simulink model "visual_line_follower_sac_lyapunov_prevlat_20260707_113326"  (R2026a)
settings: Solver=FixedStepDiscrete  StopTime=50  FixedStep=MJ_StepTime  EnableMultiTasking=on
InitFcn:
  | run(fullfile(fileparts(get_param(bdroot,"FileName")),"runtime","configure_turtlebot3_visual_line_follower_paths.m"));
model workspace (MAT data in the model file):
  BaseLinearSpeed = 20
  BaseSpeedScale = 0.03
  Kd_Line = 0.35
  Ki_Line = 0
  Kp_Line = 5
  LocalPath_CurvatureGain = 0.04
  LocalPath_HeadingGain = 0.35
  LocalPath_LateralGain = 0.6
  LocalPath_LookaheadDistance = 0.72
  LocalPath_NumPoints = 30
  LocalPath_ROIFraction = 0.1
  MJ_StepTime = 0.002
  MJ_TargetLateralPosition = 0
  MaxAngularSpeed = 1.5
  MaxWheelSpeed = 25
  N_Line = 20
  OriginBot_ErrorScale = 500
  OriginBot_MaxSaturation = 0.3
  OriginBot_MinBrightness = 70
  OriginBot_MinPixels = 30
  OriginBot_ROIHeight = 45
  OriginBot_ROIStartFraction = 0.72
  SAC_Beta = 3
  SAC_Done_Steps = 100
  SAC_Eps = 0.01
  SAC_K_inv = 0.4
  SAC_Lambda = 0.5
  SAC_MaxDeltaOmega = 1
  SAC_P_Lost = 1
  SAC_Q = 1
  SAC_Q_e = 1
  SAC_Q_h = 1
  SAC_Q_l = 1
  SAC_R = 0.1
  SteeringSign = 1
  TB3_WheelRadius = 0.033
  TB3_WheelSeparation = 0.288
  Ts_Control = 0.05
  Ts_Stop = 10
  Ts_Vision = 0.05
  TurtleBot3MuJoCoMap = "training"
  TurtleBot3MuJoCoScene = ""
undefined symbols (not defined in the file): originbot_line_follower_debug_frame, originbot_local_path_generator
libraries: mjLib x1, slpidlib x1, simulink x1, rllib x1
settings Model: ExtModeTrigDuration=10000  Creator=HP  LastModifiedBy=HP
settings SolverCC: PositivePriorityOrder=on
settings ConfigComp: CovMetricSettings=dswe

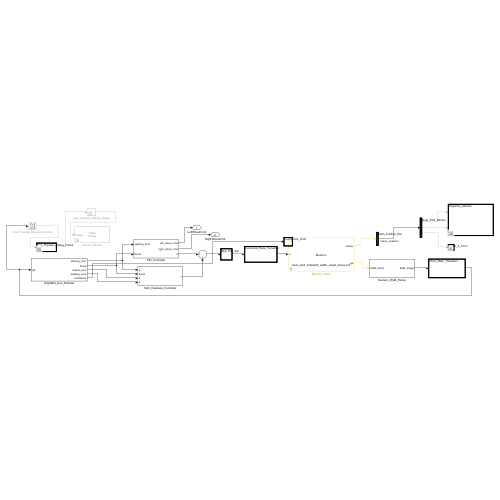
[thumbnail: Simulink's stored preview of the top-level diagram]
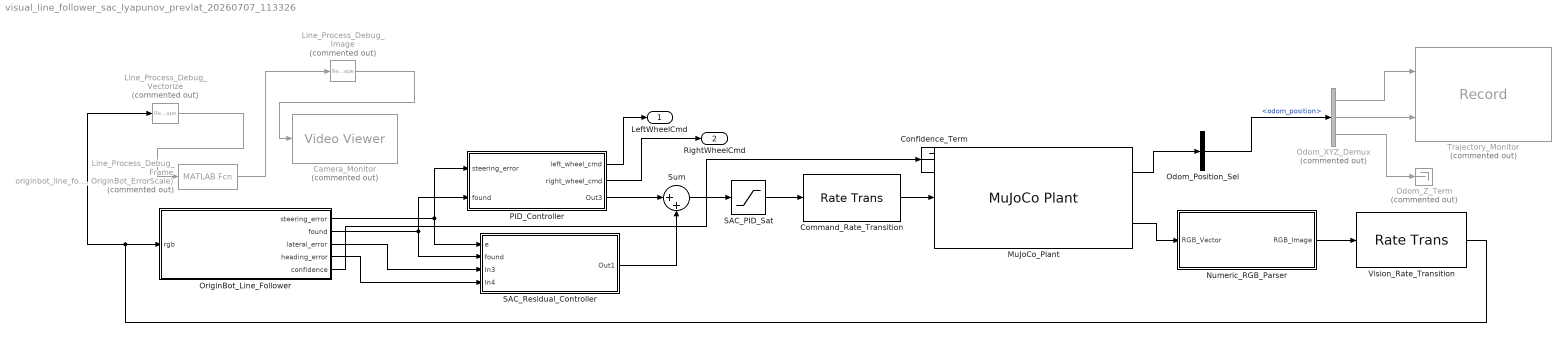
== system visual_line_follower_sac_lyapunov_prevlat_20260707_113326 ==
  Camera_Monitor : VideoViewer  Commented=on  FigPos=[498 692 990 438]
  Command_Rate_Transition : RateTransition  OutPortSampleTime=MJ_StepTime
  Confidence_Term : Terminator
  Line_Process_Debug_Frame : MATLABFcn  Commented=on  MATLABFcn=originbot_line_follower_debug_frame(u, LocalPath_ROIFraction, LocalPath_NumPoints, OriginBot_MinBrightness, OriginBot_MaxSaturation, OriginBot_MinPixels, OriginBot_ErrorScale)
  Line_Process_Debug_Image : Reshape  Commented=on  OutputDimensionality=Customize  OutputDimensions=[480,640,3]
  Line_Process_Debug_Vectorize : Reshape  Commented=on  OutputDimensionality=Column vector (2-D)
  MuJoCo_Plant : mjLib/MuJoCo Plant  controlBus=[]  sensorBus=mj_bus_sensor_7979902499018342666  controlLength=[]  sensorLength=[]  rgbLength=[]  depthLength=[]  sampleTime=0.002  xmlFileRel=D:\final_project\Sheffield\for_getting_started\src\simple_camera_pid\matlab\..\..\..\model\mujoco\turtlebot3\training_oval_track_turtlebot3_waffle_visual_scene.xml  xmlFile=D:\final_project\Sheffield\for_getting_started\src\simple_camera_pid\matlab\..\..\..\model\mujoco\turtlebot3\track_hard_turtlebot3_waffle_visual_scene.xml  renderingType=None  vsync=on  visualFPS=60  zoomLevel=1  znear=0.062275  zfar=311.3772  cameraSampleTime=Ts_Vision  rgbOutOption=on  depthOutOption=off  controlInterfaceType=Vector
      settings: SourceProductName=MuJoCo Simulator
  Numeric_RGB_Parser : Subsystem
  Odom_Position_Sel : BusSelector  OutputSignals=odom_position
  Odom_XYZ_Demux : Demux  Commented=on  Outputs=3
  Odom_Z_Term : Terminator  Commented=on
  OriginBot_Line_Follower : Subsystem
  PID_Controller : Subsystem
  SAC_PID_Sat : Saturate  UpperLimit=[MaxWheelSpeed; MaxWheelSpeed]  LowerLimit=-[MaxWheelSpeed; MaxWheelSpeed]
  SAC_Residual_Controller : Subsystem
  Sum : Sum  Inputs=|++
  Trajectory_Monitor : Record  Commented=on  NumPorts=2.0  FileSettingsInternal="{\"entries\":[{\"content\":{\"excelSettings\":{\"content\":{},\"type\":\"Streamout.ExcelSettings\"},\"parquetSettings\":{\"content\":{},\"type\":\"Streamout.ParquetSettings\"}},\"type\":\"Streamout.FileSettingStorage\",\"uuid\":\"\"}],\"packageUris\":[\"http:\\/\\/schema.mathworks.com\\/mf0\\/streamout_blocks\\/R2020a\"],\"version\":\"1.0\"}"  FrameSettings=[0, 0]  Layout=[1 1]  SignalsInternal="{\"entries\":[{\"content\":{\"signals\":[{\"content\":{\"blockPath\":[],\"dimensions\":[1,1],\"domain\":\"\",\"lineColor\":\"#a2142f\",\"plots\":[ 1 ],\"port\":1,\"signalID\":1,\"signalName\":\"Odom_XYZ_Demux:1\"},\"type\":\"RecordBlkView.Signal\",\"uuid\":\"\"},{\"content\":{\"blockPath\":[],\"dimensions\":[1,1],\"domain\":\"\",\"lineColor\":\"#139fff\",\"plots\":[ 1 ],\"port\":2,\"signalID\":2,\"signalName\":\"Odom_XYZ_Demux:2\"},\"type\":\"RecordBlkView.Signal\",\"uuid\":\"\"}]},\"type\":\"RecordBlkView.InputSignals\",\"uuid\":\"\"}],\"packageUris\":[\"http:\\/\\/schema.mathworks.com\\/mf0\\/streamout_blocks\\/R2020a\"],\"version\":\"1.0\"}"  VisualizationBindings="{\"xyplotplugin\":{\"info\":[{\"series\":[{\"bindingParametersList\":[{\"parameter\":\"X-Axis\",\"signalID\":1,\"signalName\":\"Odom_XYZ_Demux:1\"},{\"parameter\":\"Y-Axis\",\"signalID\":2,\"signalName\":\"Odom_XYZ_Demux:2\"}],\"seriesID\":0}],\"subplotID\":1}]}}"  CompatibilityTag=XY  st=-1
  Vision_Rate_Transition : RateTransition  OutPortSampleTime=Ts_Vision
  LeftWheelCmd : Outport
  RightWheelCmd : Outport  Port=2
  wires:
  Line_Process_Debug_Frame/1 -> Line_Process_Debug_Image/1
  Vision_Rate_Transition/1 -> OriginBot_Line_Follower/1(rgb), Line_Process_Debug_Vectorize/1
  PID_Controller/1(left_wheel_cmd) -> LeftWheelCmd/1
  Line_Process_Debug_Vectorize/1 -> Line_Process_Debug_Frame/1
  MuJoCo_Plant/2 -> Numeric_RGB_Parser/1(RGB_Vector)
  OriginBot_Line_Follower/2(found) -> PID_Controller/2(found), SAC_Residual_Controller/2(found)
  OriginBot_Line_Follower/1(steering_error) -> PID_Controller/1(steering_error), SAC_Residual_Controller/1(e)
  Command_Rate_Transition/1 -> MuJoCo_Plant/1
  PID_Controller/2(right_wheel_cmd) -> RightWheelCmd/1
  Line_Process_Debug_Image/1 -> Camera_Monitor/1
  Numeric_RGB_Parser/1(RGB_Image) -> Vision_Rate_Transition/1
  OriginBot_Line_Follower/3(lateral_error) -> SAC_Residual_Controller/3(In3)
  OriginBot_Line_Follower/4(heading_error) -> SAC_Residual_Controller/4(In4)
  PID_Controller/3(Out3) -> Sum/1
  SAC_Residual_Controller/1(Out1) -> Sum/2
  Sum/1 -> SAC_PID_Sat/1
  SAC_PID_Sat/1 -> Command_Rate_Transition/1
  MuJoCo_Plant/1 -> Odom_Position_Sel/1
  Odom_Position_Sel/1 -> Odom_XYZ_Demux/1  "<odom_position>"
  Odom_XYZ_Demux/1 -> Trajectory_Monitor/1
  Odom_XYZ_Demux/2 -> Trajectory_Monitor/2
  Odom_XYZ_Demux/3 -> Odom_Z_Term/1
  OriginBot_Line_Follower/5(confidence) -> Confidence_Term/1

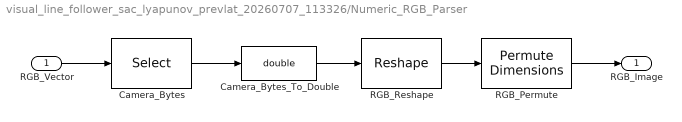
== system visual_line_follower_sac_lyapunov_prevlat_20260707_113326/Numeric_RGB_Parser ==
  RGB_Vector : Inport
  Camera_Bytes : Selector  InputPortWidth=921601  IndexOptions=Index vector (dialog)  Indices=1:921600  OutputSizes=1
  Camera_Bytes_To_Double : DataTypeConversion  OutDataTypeStr=double
  RGB_Permute : PermuteDimensions  Order=[3 2 1]
  RGB_Reshape : Reshape  OutputDimensionality=Customize  OutputDimensions=[3,640,480]
  RGB_Image : Outport
  wires:
  Camera_Bytes_To_Double/1 -> RGB_Reshape/1
  RGB_Permute/1 -> RGB_Image/1
  RGB_Reshape/1 -> RGB_Permute/1
  Camera_Bytes/1 -> Camera_Bytes_To_Double/1
  RGB_Vector/1 -> Camera_Bytes/1

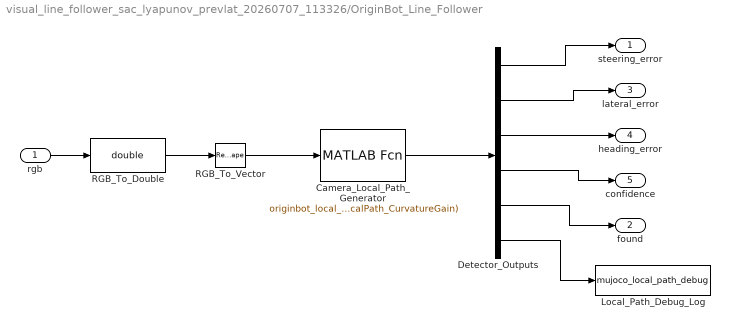
== system visual_line_follower_sac_lyapunov_prevlat_20260707_113326/OriginBot_Line_Follower ==
  rgb : Inport
  Camera_Local_Path_Generator : MATLABFcn  MATLABFcn=originbot_local_path_generator(u, LocalPath_ROIFraction, LocalPath_NumPoints, OriginBot_MinBrightness, OriginBot_MaxSaturation, OriginBot_MinPixels, OriginBot_ErrorScale, LocalPath_LookaheadDistance, LocalPath_LateralGain, LocalPath_HeadingGain, LocalPath_CurvatureGain)  OutputDimensions=72  OutputSignalType=real  SampleTime=Ts_Vision
  Detector_Outputs : Demux  Outputs=[1 1 1 1 1 67]
  Local_Path_Debug_Log : ToWorkspace  VariableName=mujoco_local_path_debug  SaveFormat=Timeseries  SampleTime=-1
  RGB_To_Double : DataTypeConversion  OutDataTypeStr=double
  RGB_To_Vector : Reshape  OutputDimensionality=Column vector (2-D)
  steering_error : Outport
  found : Outport  Port=2
  lateral_error : Outport  Port=3
  heading_error : Outport  Port=4
  confidence : Outport  Port=5
  wires:
  Detector_Outputs/2 -> lateral_error/1
  rgb/1 -> RGB_To_Double/1
  RGB_To_Double/1 -> RGB_To_Vector/1
  RGB_To_Vector/1 -> Camera_Local_Path_Generator/1
  Detector_Outputs/4 -> confidence/1
  Camera_Local_Path_Generator/1 -> Detector_Outputs/1
  Detector_Outputs/1 -> steering_error/1
  Detector_Outputs/3 -> heading_error/1
  Detector_Outputs/5 -> found/1
  Detector_Outputs/6 -> Local_Path_Debug_Log/1

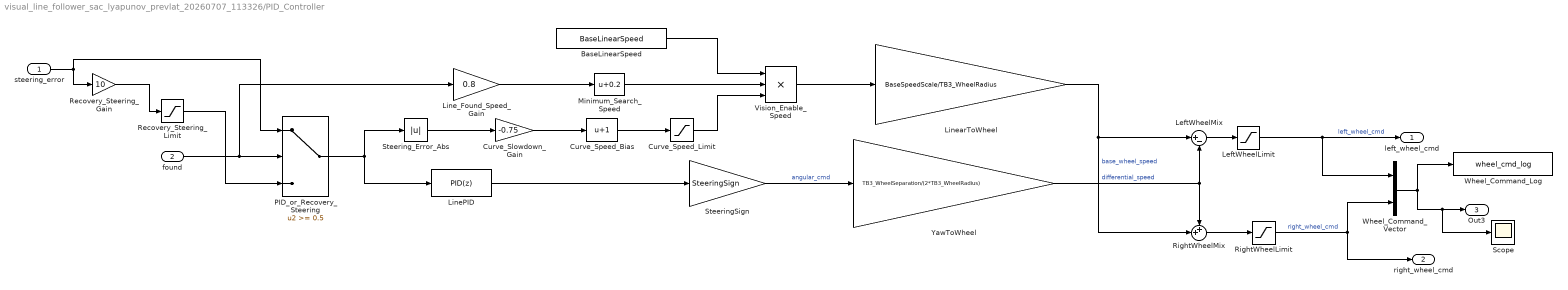
== system visual_line_follower_sac_lyapunov_prevlat_20260707_113326/PID_Controller ==
  steering_error : Inport
  found : Inport  Port=2
  BaseLinearSpeed : Constant  Value=BaseLinearSpeed
  Curve_Slowdown_Gain : Gain  Gain=-0.75
  Curve_Speed_Bias : Bias  Bias=1
  Curve_Speed_Limit : Saturate  UpperLimit=1  LowerLimit=0.25
  LeftWheelLimit : Saturate  UpperLimit=MaxWheelSpeed  LowerLimit=-MaxWheelSpeed
  LeftWheelMix : Sum  Inputs=|+-
  LinePID : slpidlib/PID Controller  Controller=PID  Form=Parallel  TimeDomain=Discrete-time  UseExternalTs=off  SampleTime=Ts_Control  IntegratorMethod=Backward Euler  FilterMethod=Trapezoidal  ControllerParametersSource=internal  P=Kp_Line  I=Ki_Line  UseKiTs=off  D=Kd_Line  UseExternalDerivativeSource=off  N=N_Line  UseFilter=on  TunerSelectOption=Transfer Function Based (PID Tuner App)  InitialConditionSource=internal  InitialConditionForIntegrator=0  InitialConditionForFilter=0  DifferentiatorICPrevScaledInput=0  ExternalReset=none  TrackingMode=off  Kt=1  LimitOutput=on  SatLimitsSource=internal  UpperSaturationLimit=MaxAngularSpeed  LowerSaturationLimit=-MaxAngularSpeed  LinearizeAsGain=off  AntiWindupMode=back-calculation  Kb=1  LimitIntegrator=off  UpperIntegratorSaturationLimit=inf  LowerIntegratorSaturationLimit=-inf  POutMin=[]  POutMax=[]  IOutMin=[]  IOutMax=[]  DOutMin=[]  DOutMax=[]  NOutMin=[]  NOutMax=[]  SumOutMin=[]  SumOutMax=[]  SaturationOutMin=[]  SaturationOutMax=[]  PParamMin=[]  PParamMax=[]  IParamMin=[]  IParamMax=[]  DParamMin=[]  DParamMax=[]  NParamMin=[]  NParamMax=[]  KbParamMin=[]  KbParamMax=[]  KtParamMin=[]  KtParamMax=[]  KbOutMin=[]  KbOutMax=[]  KtOutMin=[]  KtOutMax=[]  IntegratorOutMin=[]  IntegratorOutMax=[]  FilterOutMin=[]  FilterOutMax=[]  SumI1OutMin=[]  SumI1OutMax=[]  SumI2OutMin=[]  SumI2OutMax=[]  SumI3OutMin=[]  SumI3OutMax=[]  SumI4OutMin=[]  SumI4OutMax=[]  SumDOutMin=[]  SumDOutMax=[]  DifferentiatorOutMin=[]  DifferentiatorOutMax=[]  FilterDiffOutCoefMin=[]  FilterDiffOutCoefMax=[]  ReciprocalOutMin=[]  ReciprocalOutMax=[]  SumDenOutMin=[]  SumDenOutMax=[]  SumNumOutMin=[]  SumNumOutMax=[]  DivideOutMin=[]  DivideOutMax=[]  UdiffTsProdOutMin=[]  UdiffTsProdOutMax=[]  NTsProdOutMin=[]  NTsProdOutMax=[]  UintegralTsProdOutMin=[]  UintegralTsProdOutMax=[]  UngainTsProdOutMin=[]  UngainTsProdOutMax=[]  ClampingZeroOutDataTypeStr=Inherit: Inherit via back propagation  ClampingZeroOutMin=[]  ClampingZeroOutMax=[]  FilterDenConstantOutDataTypeStr=Inherit: Inherit via back propagation  FilterDenConstantOutMin=[]  FilterDenConstantOutMax=[]  PCopyOutDataTypeStr=Inherit: Inherit via back propagation  PCopyOutMin=[]  PCopyOutMax=[]  NCopyOutDataTypeStr=Inherit: Inherit via back propagation  NCopyOutMin=[]  NCopyOutMax=[]  IntegratorContinuousStateAttributes=''  IntegratorStateMustResolveToSignalObject=off  IntegratorRTWStateStorageClass=Auto  FilterContinuousStateAttributes=''  FilterStateMustResolveToSignalObject=off  FilterRTWStateStorageClass=Auto  ParallelPVariant=InternalParameters  IdealPVariant=Disabled  IVariant=InternalParameters  DVariant=InternalParameters  IntegratorVariant=Discrete  SatVariant=Enabled  AWVariant=BackCalculation  PCopyVariant=Disabled  TRVariant=Disabled  FdbkBlocksVariant=Feedback  IdealPFdbkVariant=Passthrough  SatFdbkVariant=Enabled  DerivativeFilterVariant=TrapezoidalFilter  NVariant=InternalParameters  NCopyVariant=InternalParameters  FilterICVariant=InternalICsFilter  IntegratorICVariant=InternalICs  ExternalResetVariant=Disabled  TRSumVariant=Passthrough  SumFdbkVariant=Enabled  SumVariant=Sum_PID  TsampFilterVariant=InternalTs  TsampNgainVariant=Passthrough  TsampIntegralVariant=Disabled_SignalSpec  ExternalSaturationOutDataTypeStr=Inherit: Same as second input  DerivativeSourceVariant=ErrorSignal  PreIntVariant=InternalPreInt
      settings: LibrarySourceBlock=hdlsllib/Discrete/Discrete PID Controller
  Line_Found_Speed_Gain : Gain  Gain=0.8
  LinearToWheel : Gain  Gain=BaseSpeedScale/TB3_WheelRadius
  Minimum_Search_Speed : Bias  Bias=0.2
  PID_or_Recovery_Steering : Switch  Threshold=0.5
  Recovery_Steering_Gain : Gain  Gain=10
  Recovery_Steering_Limit : Saturate  UpperLimit=0.45  LowerLimit=-0.45
  RightWheelLimit : Saturate  UpperLimit=MaxWheelSpeed  LowerLimit=-MaxWheelSpeed
  RightWheelMix : Sum  Inputs=++|
  Scope : Scope
  SteeringSign : Gain  Gain=SteeringSign
  Steering_Error_Abs : Abs
  Vision_Enable_Speed : Product  Inputs=***
  Wheel_Command_Log : ToWorkspace  VariableName=wheel_cmd_log  SaveFormat=Structure With Time
  Wheel_Command_Vector : Mux  Inputs=2
  YawToWheel : Gain  Gain=TB3_WheelSeparation/(2*TB3_WheelRadius)
  left_wheel_cmd : Outport
  right_wheel_cmd : Outport  Port=2
  Out3 : Outport  Port=3
  wires:
  LeftWheelLimit/1 -> Wheel_Command_Vector/1, left_wheel_cmd/1  "left_wheel_cmd"
  steering_error/1 -> Recovery_Steering_Gain/1, PID_or_Recovery_Steering/1
  Minimum_Search_Speed/1 -> Vision_Enable_Speed/2
  found/1 -> Line_Found_Speed_Gain/1, PID_or_Recovery_Steering/2
  PID_or_Recovery_Steering/1 -> Steering_Error_Abs/1, LinePID/1
  Recovery_Steering_Gain/1 -> Recovery_Steering_Limit/1
  Recovery_Steering_Limit/1 -> PID_or_Recovery_Steering/3
  Line_Found_Speed_Gain/1 -> Minimum_Search_Speed/1
  Steering_Error_Abs/1 -> Curve_Slowdown_Gain/1
  Curve_Slowdown_Gain/1 -> Curve_Speed_Bias/1
  Curve_Speed_Bias/1 -> Curve_Speed_Limit/1
  LinePID/1 -> SteeringSign/1
  BaseLinearSpeed/1 -> Vision_Enable_Speed/1
  Curve_Speed_Limit/1 -> Vision_Enable_Speed/3
  Vision_Enable_Speed/1 -> LinearToWheel/1
  SteeringSign/1 -> YawToWheel/1  "angular_cmd"
  LinearToWheel/1 -> LeftWheelMix/1, RightWheelMix/2  "base_wheel_speed"
  YawToWheel/1 -> RightWheelMix/1, LeftWheelMix/2  "differential_speed"
  LeftWheelMix/1 -> LeftWheelLimit/1
  RightWheelMix/1 -> RightWheelLimit/1
  RightWheelLimit/1 -> right_wheel_cmd/1, Wheel_Command_Vector/2  "right_wheel_cmd"
  Wheel_Command_Vector/1 -> Scope/1, Out3/1, Wheel_Command_Log/1

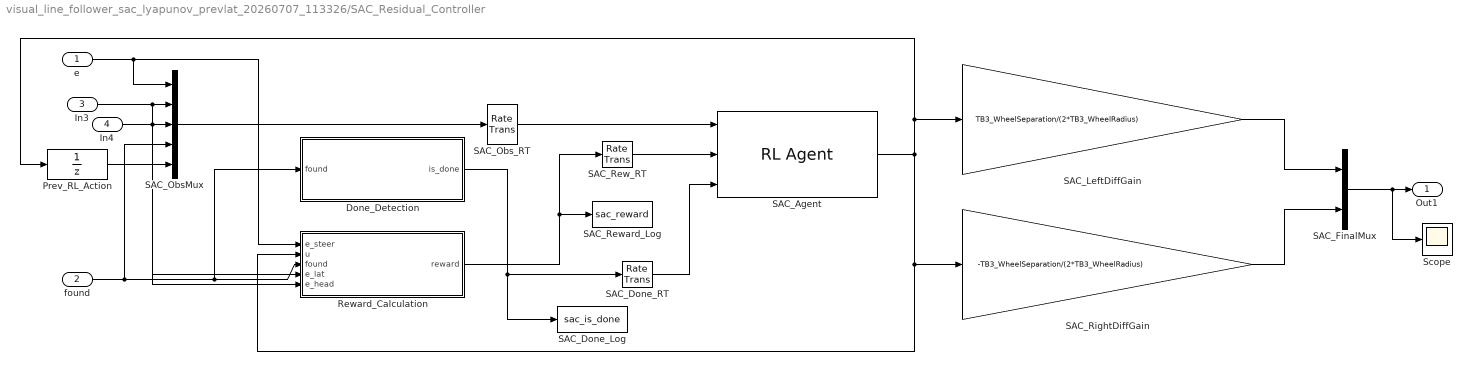
== system visual_line_follower_sac_lyapunov_prevlat_20260707_113326/SAC_Residual_Controller ==
  e : Inport
  found : Inport  Port=2
  In3 : Inport  Port=3
  In4 : Inport  Port=4
  Done_Detection : Subsystem
  Prev_RL_Action : UnitDelay  SampleTime=Ts_Control
  Reward_Calculation : Subsystem
  SAC_Agent : rllib/RL Agent  Agent=agent  ExternalActionAsInput=off  ProvideLastAction=off  ProvideCumRwd=off  TreatAsDirectFeedthrough=on  UseStrictObservationDataTypes=off
  SAC_Done_Log : ToWorkspace  VariableName=sac_is_done  SaveFormat=Timeseries  SampleTime=-1
  SAC_Done_RT : RateTransition  Integrity=off  Deterministic=off
  SAC_FinalMux : Mux  Inputs=2
  SAC_LeftDiffGain : Gain  Gain=TB3_WheelSeparation/(2*TB3_WheelRadius)
  SAC_ObsMux : Mux  Inputs=5
  SAC_Obs_RT : RateTransition  Integrity=off  Deterministic=off
  SAC_Rew_RT : RateTransition  Integrity=off  Deterministic=off
  SAC_Reward_Log : ToWorkspace  VariableName=sac_reward  SaveFormat=Timeseries  SampleTime=-1
  SAC_RightDiffGain : Gain  Gain=-TB3_WheelSeparation/(2*TB3_WheelRadius)
  Scope : Scope
      settings: ActiveDisplayYMinimum=-1  ActiveDisplayYMaximum=1
  Out1 : Outport
  wires:
  e/1 -> Reward_Calculation/1(e_steer), SAC_ObsMux/1
  found/1 -> Done_Detection/1(found), Reward_Calculation/3(found), SAC_ObsMux/4
  SAC_Rew_RT/1 -> SAC_Agent/2
  SAC_Done_RT/1 -> SAC_Agent/3
  SAC_Obs_RT/1 -> SAC_Agent/1
  SAC_Agent/1 -> Reward_Calculation/2(u), SAC_RightDiffGain/1, Prev_RL_Action/1, SAC_LeftDiffGain/1
  In3/1 -> SAC_ObsMux/2, Reward_Calculation/4(e_lat)
  In4/1 -> SAC_ObsMux/3, Reward_Calculation/5(e_head)
  Prev_RL_Action/1 -> SAC_ObsMux/5
  SAC_ObsMux/1 -> SAC_Obs_RT/1
  SAC_LeftDiffGain/1 -> SAC_FinalMux/1
  SAC_RightDiffGain/1 -> SAC_FinalMux/2
  SAC_FinalMux/1 -> Scope/1, Out1/1
  Reward_Calculation/1(reward) -> SAC_Rew_RT/1, SAC_Reward_Log/1
  Done_Detection/1(is_done) -> SAC_Done_Log/1, SAC_Done_RT/1

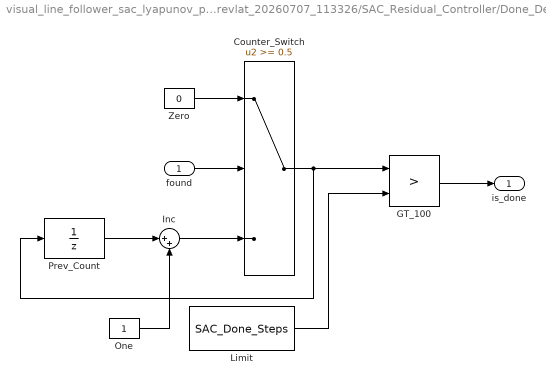
== system visual_line_follower_sac_lyapunov_prevlat_20260707_113326/SAC_Residual_Controller/Done_Detection ==
  found : Inport
  Counter_Switch : Switch  Threshold=0.5  SaturateOnIntegerOverflow=off  InputSameDT=off
  GT_100 : RelationalOperator  Operator=>  OutDataTypeStr=boolean  RndMeth=Simplest  InputSameDT=off
  Inc : Sum  Inputs=|++
  Limit : Constant  Value=SAC_Done_Steps
  One : Constant
  Prev_Count : UnitDelay  SampleTime=Ts_Control
  Zero : Constant  Value=0
  is_done : Outport
  wires:
  Prev_Count/1 -> Inc/1
  One/1 -> Inc/2
  found/1 -> Counter_Switch/2
  Zero/1 -> Counter_Switch/1
  GT_100/1 -> is_done/1
  Inc/1 -> Counter_Switch/3
  Limit/1 -> GT_100/2
  Counter_Switch/1 -> Prev_Count/1, GT_100/1

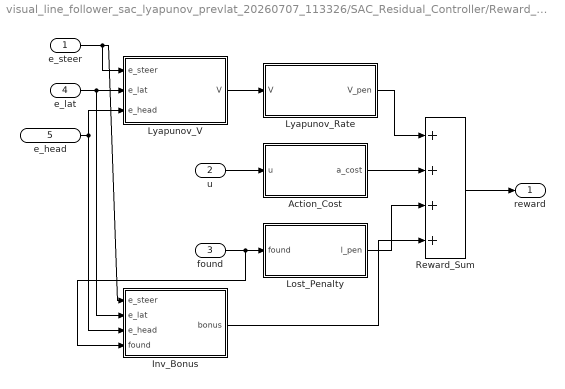
== system visual_line_follower_sac_lyapunov_prevlat_20260707_113326/SAC_Residual_Controller/Reward_Calculation ==
  e_steer : Inport
  u : Inport  Port=2
  found : Inport  Port=3
  e_lat : Inport  Port=4
  e_head : Inport  Port=5
  Action_Cost : Subsystem
  Inv_Bonus : Subsystem
  Lost_Penalty : Subsystem
  Lyapunov_Rate : Subsystem
  Lyapunov_V : Subsystem
  Reward_Sum : Sum  Inputs=++++
  reward : Outport
  wires:
  found/1 -> Inv_Bonus/4(found), Lost_Penalty/1(found)
  u/1 -> Action_Cost/1(u)
  e_steer/1 -> Lyapunov_V/1(e_steer), Inv_Bonus/1(e_steer)
  e_head/1 -> Lyapunov_V/3(e_head), Inv_Bonus/3(e_head)
  e_lat/1 -> Lyapunov_V/2(e_lat), Inv_Bonus/2(e_lat)
  Lyapunov_V/1(V) -> Lyapunov_Rate/1(V)
  Inv_Bonus/1(bonus) -> Reward_Sum/4
  Lyapunov_Rate/1(V_pen) -> Reward_Sum/1
  Action_Cost/1(a_cost) -> Reward_Sum/2
  Lost_Penalty/1(l_pen) -> Reward_Sum/3
  Reward_Sum/1 -> reward/1

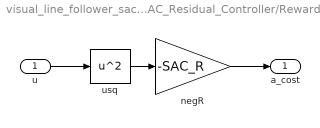
== system visual_line_follower_sac_lyapunov_prevlat_20260707_113326/SAC_Residual_Controller/Reward_Calculation/Action_Cost ==
  u : Inport
  negR : Gain  Gain=-SAC_R
  usq : Math  Operator=square
  a_cost : Outport
  wires:
  u/1 -> usq/1
  usq/1 -> negR/1
  negR/1 -> a_cost/1

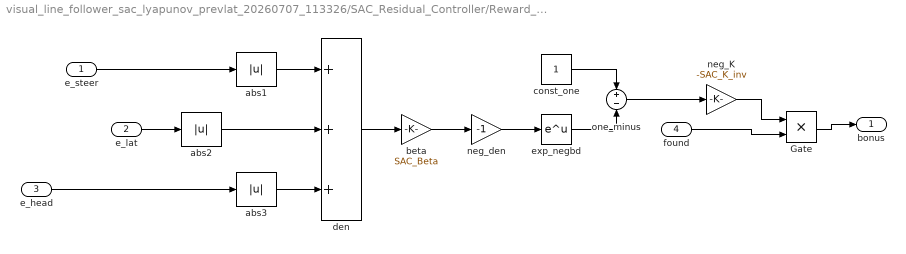
== system visual_line_follower_sac_lyapunov_prevlat_20260707_113326/SAC_Residual_Controller/Reward_Calculation/Inv_Bonus ==
  e_steer : Inport
  e_lat : Inport  Port=2
  e_head : Inport  Port=3
  found : Inport  Port=4
  Gate : Product
  abs1 : Abs  SaturateOnIntegerOverflow=off
  abs2 : Abs  SaturateOnIntegerOverflow=off
  abs3 : Abs  SaturateOnIntegerOverflow=off
  beta : Gain  Gain=SAC_Beta
  const_one : Constant
  den : Sum  Inputs=+++
  exp_negbd : Math
  neg_K : Gain  Gain=-SAC_K_inv
  neg_den : Gain  Gain=-1
  one_minus : Sum  Inputs=+-
  bonus : Outport
  wires:
  neg_K/1 -> Gate/1
  one_minus/1 -> neg_K/1
  exp_negbd/1 -> one_minus/2
  const_one/1 -> one_minus/1
  neg_den/1 -> exp_negbd/1
  beta/1 -> neg_den/1
  den/1 -> beta/1
  Gate/1 -> bonus/1
  found/1 -> Gate/2
  e_steer/1 -> abs1/1
  e_lat/1 -> abs2/1
  e_head/1 -> abs3/1
  abs1/1 -> den/1
  abs3/1 -> den/3
  abs2/1 -> den/2

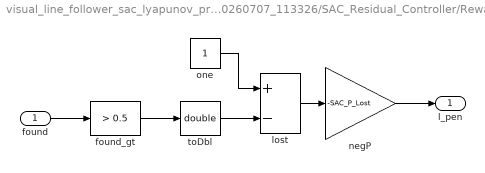
== system visual_line_follower_sac_lyapunov_prevlat_20260707_113326/SAC_Residual_Controller/Reward_Calculation/Lost_Penalty ==
  found : Inport
  found_gt : simulink/Logic and Bit Operations/Compare To Constant  relop=>  const=0.5  OutDataTypeStr=boolean
  lost : Sum  Inputs=+-
  negP : Gain  Gain=-SAC_P_Lost
  one : Constant
  toDbl : DataTypeConversion  OutDataTypeStr=double  SaturateOnIntegerOverflow=off  RndMeth=Floor
  l_pen : Outport
  wires:
  negP/1 -> l_pen/1
  toDbl/1 -> lost/2
  found/1 -> found_gt/1
  lost/1 -> negP/1
  one/1 -> lost/1
  found_gt/1 -> toDbl/1

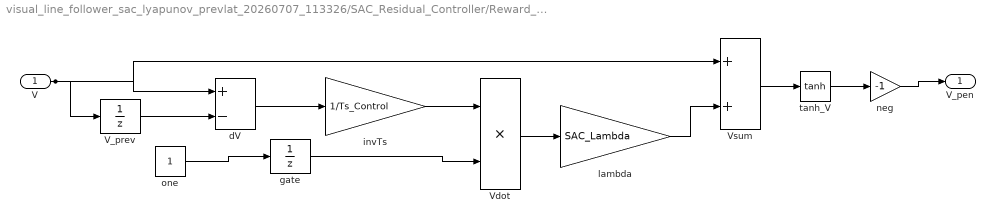
== system visual_line_follower_sac_lyapunov_prevlat_20260707_113326/SAC_Residual_Controller/Reward_Calculation/Lyapunov_Rate ==
  V : Inport
  V_prev : UnitDelay  SampleTime=Ts_Control
  Vdot : Product
  Vsum : Sum
  dV : Sum  Inputs=+-
  gate : UnitDelay  SampleTime=Ts_Control
  invTs : Gain  Gain=1/Ts_Control
  lambda : Gain  Gain=SAC_Lambda
  neg : Gain  Gain=-1
  one : Constant  SampleTime=Ts_Control
  tanh_V : Trigonometry  Operator=tanh
  V_pen : Outport
  wires:
  tanh_V/1 -> neg/1
  Vsum/1 -> tanh_V/1
  V/1 -> V_prev/1, Vsum/1, dV/1
  V_prev/1 -> dV/2
  dV/1 -> invTs/1
  Vdot/1 -> lambda/1
  one/1 -> gate/1
  invTs/1 -> Vdot/1
  lambda/1 -> Vsum/2
  gate/1 -> Vdot/2
  neg/1 -> V_pen/1

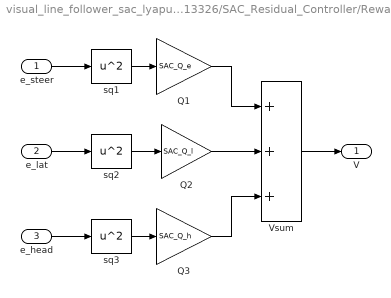
== system visual_line_follower_sac_lyapunov_prevlat_20260707_113326/SAC_Residual_Controller/Reward_Calculation/Lyapunov_V ==
  e_steer : Inport
  e_lat : Inport  Port=2
  e_head : Inport  Port=3
  Q1 : Gain  Gain=SAC_Q_e
  Q2 : Gain  Gain=SAC_Q_l
  Q3 : Gain  Gain=SAC_Q_h
  Vsum : Sum  Inputs=+++
  sq1 : Math  Operator=square
  sq2 : Math  Operator=square
  sq3 : Math  Operator=square
  V : Outport
  wires:
  Q1/1 -> Vsum/1
  e_steer/1 -> sq1/1
  sq1/1 -> Q1/1
  e_lat/1 -> sq2/1
  sq3/1 -> Q3/1
  e_head/1 -> sq3/1
  sq2/1 -> Q2/1
  Q2/1 -> Vsum/2
  Q3/1 -> Vsum/3
  Vsum/1 -> V/1
